simulink model "TrajectoryTracking_2015b_00"  (R2017a)
settings: Solver=ode45  StartTime=0.0  StopTime=125  RelTol=1e-3
values from neighbouring files (symbols this model uses):
  B_input = B_T    [ErrorDynamicsControllerDesign.m]
  tau_d_1 = C_RB1+C_A1+D1+G1    [DesiredInputOptimalConfiguration.m]
  tau_d_2 = C_RB2+C_A2+D2+G2    [DesiredInputOptimalConfiguration.m]
undefined symbols (not defined in the file or in its folder): angular_velocity_pitch_1, angular_velocity_pitch_2, angular_velocity_roll_1, angular_velocity_roll_2, angular_velocity_yaw_1, angular_velocity_yaw_2, K1, K2, linear_velocity_x_1, linear_velocity_x_2, linear_velocity_y_1, linear_velocity_y_2, linear_velocity_z_1, linear_velocity_z_2, pitch_angle_1, pitch_angle_2, roll_angle_1, roll_angle_2, t_1_last, t_e_1, t_e_2, tau_d_3, tau_d_4, tau_d_5, tau_d_6, tau_d_7, u_d_1, u_d_2, u_d_optimized, veh, x1, x2, y1, y2, yaw_angle_1, yaw_angle_2, z1, z2
undefined symbols (not defined in the file): b_T1_optimized, b_T2_optimized, b_T3_optimized, b_T4_optimized, b_T5_optimized, b_T6_optimized, d_T1_optimized, d_T2_optimized, d_T3_optimized, d_T4_optimized, d_T5_optimized, d_T6_optimized, r_T1_optimized, r_T2_optimized, r_T3_optimized, r_T4_optimized, r_T5_optimized, r_T6_optimized
libraries: sharedtransform x1, shared6dofsys x1
(part 2 of 2)

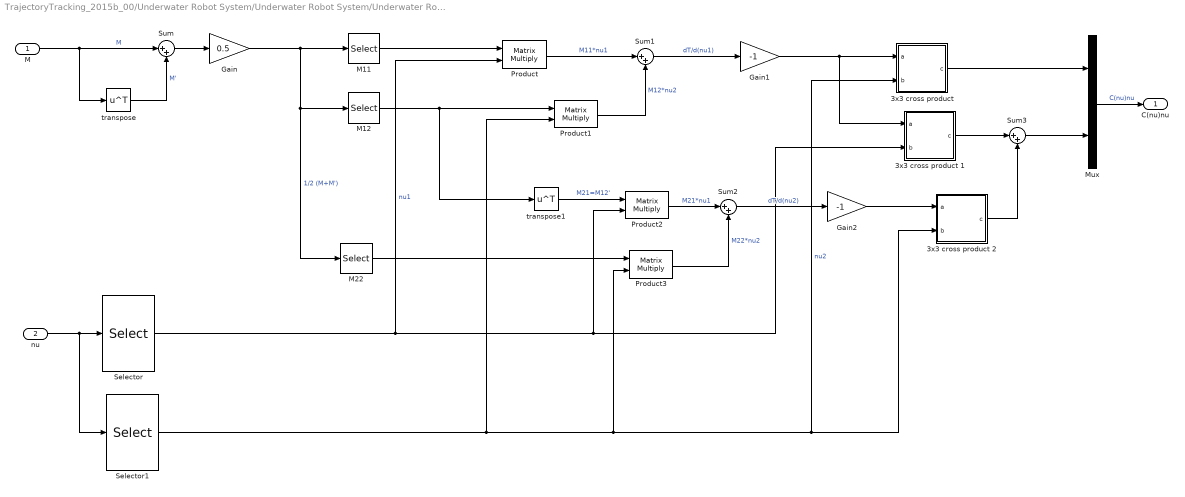
== system TrajectoryTracking_2015b_00/Underwater Robot System/Underwater Robot System/Underwater Robot Dynamics /6DOF Coriolis forces ==
  M : Inport
  nu : Inport  Port=2
  3x3 cross product : Subsystem
  3x3 cross product 1 : Subsystem
  3x3 cross product 2 : Subsystem
  Gain : Gain  Gain=0.5  SaturateOnIntegerOverflow=on  OutDataTypeStr=Inherit: Same as input  ParamDataTypeStr=Inherit: Same as input
  Gain1 : Gain  Gain=-1  SaturateOnIntegerOverflow=on  OutDataTypeStr=Inherit: Same as input  ParamDataTypeStr=Inherit: Same as input
  Gain2 : Gain  Gain=-1  SaturateOnIntegerOverflow=on  OutDataTypeStr=Inherit: Same as input  ParamDataTypeStr=Inherit: Same as input
  M11 : Selector  NumberOfDimensions=2  InputPortWidth=3  IndexOptions=Index vector (dialog),Index vector (dialog)  Indices=[1 2 3],[1 2 3]  OutputSizes=1
  M12 : Selector  NumberOfDimensions=2  InputPortWidth=3  IndexOptions=Index vector (dialog),Index vector (dialog)  Indices=[1 2 3],[4 5 6]  OutputSizes=1
  M22 : Selector  NumberOfDimensions=2  InputPortWidth=3  IndexOptions=Index vector (dialog),Index vector (dialog)  Indices=[4 5 6],[4 5 6]  OutputSizes=1
  Mux : Mux  Inputs=2
  Product{,1..3} (4 alike) : Product  Multiplication=Matrix(*)  SaturateOnIntegerOverflow=on  OutDataTypeStr=Inherit: Same as first input
  Selector : Selector  InputPortWidth=6  IndexOptions=Index vector (dialog)  Indices=[1 2 3]  OutputSizes=1
  Selector1 : Selector  InputPortWidth=6  IndexOptions=Index vector (dialog)  Indices=[4 5 6]  OutputSizes=1
  Sum{,1..3} (4 alike) : Sum  Inputs=|++  SaturateOnIntegerOverflow=on
  transpose : Math  Operator=transpose  SaturateOnIntegerOverflow=on
  transpose1 : Math  Operator=transpose  SaturateOnIntegerOverflow=on
  C(nu)nu : Outport
  wires:
  transpose/1 -> Sum/2  "M'"
  Sum/1 -> Gain/1
  Gain/1 -> M22/1, M12/1, M11/1  "1/2 (M+M')"
  Selector/1 -> Product2/2, 3x3 cross product 1/2(b), Product/2  "nu1"
  Selector1/1 -> 3x3 cross product/2(b), 3x3 cross product 2/2(b), Product3/2, Product1/2  "nu2"
  M11/1 -> Product/1
  Product/1 -> Sum1/1  "M11*nu1"
  M12/1 -> transpose1/1, Product1/1
  Product1/1 -> Sum1/2  "M12*nu2"
  Sum1/1 -> Gain1/1  "dT/d(nu1)"
  transpose1/1 -> Product2/1  "M21=M12'"
  Product2/1 -> Sum2/1  "M21*nu1"
  M22/1 -> Product3/1
  Product3/1 -> Sum2/2  "M22*nu2"
  Sum2/1 -> Gain2/1  "dT/d(nu2)"
  Gain1/1 -> 3x3 cross product/1(a), 3x3 cross product 1/1(a)
  3x3 cross product/1(c) -> Mux/1
  Gain2/1 -> 3x3 cross product 2/1(a)
  3x3 cross product 1/1(c) -> Sum3/1
  3x3 cross product 2/1(c) -> Sum3/2
  Sum3/1 -> Mux/2
  Mux/1 -> C(nu)nu/1  "C(nu)nu"
  nu/1 -> Selector/1, Selector1/1
  M/1 -> transpose/1, Sum/1  "M"

== system TrajectoryTracking_2015b_00/Nonlinear Transformation/Position Error /Nonlinear Orientation Transformation/pitch_error/theta_d ==
  SwitchSchedule : Inport
  1-D Lookup Table1 : Lookup_n-D  NumberOfTableDimensions=1  BreakpointsForDimension1=t_e_2  Table=pitch_angle_2  InternalRulePriority=Speed  RndMeth=Simplest  InputSameDT=on
  1-D Lookup Table3 : Lookup_n-D  NumberOfTableDimensions=1  BreakpointsForDimension1=t_e_1  Table=pitch_angle_1  InternalRulePriority=Speed  RndMeth=Simplest  InputSameDT=on
  Add : Sum  Inputs=+-
  Clock : Clock
  Constant : Constant  Value=t_1_last
  Multiport Switch1 : MultiPortSwitch  Inputs=2
  Transfer Fcn : TransferFcn  Denominator=[1.5 1]
  theta_d : Outport
  wires:
  SwitchSchedule/1 -> Multiport Switch1/1
  1-D Lookup Table1/1 -> Multiport Switch1/3
  1-D Lookup Table3/1 -> Multiport Switch1/2
  Constant/1 -> Add/2
  Multiport Switch1/1 -> Transfer Fcn/1
  Clock/1 -> Add/1, 1-D Lookup Table3/1
  Add/1 -> 1-D Lookup Table1/1
  Transfer Fcn/1 -> theta_d/1

== system TrajectoryTracking_2015b_00/Nonlinear Transformation/Position Error /Nonlinear Orientation Transformation/roll_error/phi_d ==
  SwitchSchedule : Inport
  1-D Lookup Table1 : Lookup_n-D  NumberOfTableDimensions=1  BreakpointsForDimension1=t_e_2  Table=roll_angle_2  InternalRulePriority=Speed  RndMeth=Simplest  InputSameDT=on
  1-D Lookup Table3 : Lookup_n-D  NumberOfTableDimensions=1  BreakpointsForDimension1=t_e_1  Table=roll_angle_1  InternalRulePriority=Speed  RndMeth=Simplest  InputSameDT=on
  Add : Sum  Inputs=+-
  Clock : Clock
  Constant : Constant  Value=t_1_last
  Multiport Switch : MultiPortSwitch  Inputs=2
  Transfer Fcn : TransferFcn  Denominator=[1 1]
  phi_d : Outport
  wires:
  1-D Lookup Table1/1 -> Multiport Switch/3
  1-D Lookup Table3/1 -> Multiport Switch/2
  Constant/1 -> Add/2
  Multiport Switch/1 -> Transfer Fcn/1
  Clock/1 -> Add/1, 1-D Lookup Table3/1
  Add/1 -> 1-D Lookup Table1/1
  SwitchSchedule/1 -> Multiport Switch/1
  Transfer Fcn/1 -> phi_d/1

== system TrajectoryTracking_2015b_00/Nonlinear Transformation/Position Error /Nonlinear Orientation Transformation/yaw_error/theta_d ==
  SwitchSchedule : Inport
  1-D Lookup Table1 : Lookup_n-D  NumberOfTableDimensions=1  BreakpointsForDimension1=t_e_2  Table=yaw_angle_2  InternalRulePriority=Speed  RndMeth=Simplest  InputSameDT=on
  1-D Lookup Table3 : Lookup_n-D  NumberOfTableDimensions=1  BreakpointsForDimension1=t_e_1  Table=yaw_angle_1  InternalRulePriority=Speed  RndMeth=Simplest  InputSameDT=on
  Add : Sum  Inputs=+-
  Clock : Clock
  Constant : Constant  Value=t_1_last
  Multiport Switch1 : MultiPortSwitch  Inputs=2
  Transfer Fcn : TransferFcn  Denominator=[1 1]
  yaw_d : Outport
  wires:
  SwitchSchedule/1 -> Multiport Switch1/1
  1-D Lookup Table1/1 -> Multiport Switch1/3
  1-D Lookup Table3/1 -> Multiport Switch1/2
  Constant/1 -> Add/2
  Multiport Switch1/1 -> Transfer Fcn/1
  Clock/1 -> Add/1, 1-D Lookup Table3/1
  Add/1 -> 1-D Lookup Table1/1
  Transfer Fcn/1 -> yaw_d/1

== system TrajectoryTracking_2015b_00/Nonlinear Transformation/Position Error /Nonlinear Position Transformation/x_error/x_d ==
  SwitchSchedule : Inport
  1-D Lookup Table7 : Lookup_n-D  NumberOfTableDimensions=1  BreakpointsForDimension1=t_e_2  Table=x2  InternalRulePriority=Speed  RndMeth=Simplest  InputSameDT=on
  1-D Lookup Table9 : Lookup_n-D  NumberOfTableDimensions=1  BreakpointsForDimension1=t_e_1  Table=x1  InternalRulePriority=Speed  RndMeth=Simplest  InputSameDT=on
  Add : Sum  Inputs=+-
  Clock : Clock
  Constant : Constant  Value=t_1_last
  Multiport Switch1 : MultiPortSwitch  Inputs=2
  Transfer Fcn1 : TransferFcn  Denominator=[1 1]
  x_d : Outport
  wires:
  1-D Lookup Table7/1 -> Multiport Switch1/3
  1-D Lookup Table9/1 -> Multiport Switch1/2
  Constant/1 -> Add/2
  Multiport Switch1/1 -> Transfer Fcn1/1
  SwitchSchedule/1 -> Multiport Switch1/1
  Add/1 -> 1-D Lookup Table7/1
  Transfer Fcn1/1 -> x_d/1
  Clock/1 -> Add/1, 1-D Lookup Table9/1

== system TrajectoryTracking_2015b_00/Nonlinear Transformation/Position Error /Nonlinear Position Transformation/y_error/y_d ==
  SwitchSchedule : Inport
  1-D Lookup Table10 : Lookup_n-D  NumberOfTableDimensions=1  BreakpointsForDimension1=t_e_1  Table=y1  InternalRulePriority=Speed  RndMeth=Simplest  InputSameDT=on
  1-D Lookup Table8 : Lookup_n-D  NumberOfTableDimensions=1  BreakpointsForDimension1=t_e_2  Table=y2  InternalRulePriority=Speed  RndMeth=Simplest  InputSameDT=on
  Add : Sum  Inputs=+-
  Clock : Clock
  Constant : Constant  Value=t_1_last
  Multiport Switch : MultiPortSwitch  Inputs=2
  Transfer Fcn : TransferFcn  Denominator=[1 1]
  y_d : Outport
  wires:
  1-D Lookup Table8/1 -> Multiport Switch/3
  1-D Lookup Table10/1 -> Multiport Switch/2
  Constant/1 -> Add/2
  Multiport Switch/1 -> Transfer Fcn/1
  Add/1 -> 1-D Lookup Table8/1
  SwitchSchedule/1 -> Multiport Switch/1
  Clock/1 -> Add/1, 1-D Lookup Table10/1
  Transfer Fcn/1 -> y_d/1

== system TrajectoryTracking_2015b_00/Nonlinear Transformation/Position Error /Nonlinear Position Transformation/z_error/z_d ==
  SwitchSchedule : Inport
  1-D Lookup Table1 : Lookup_n-D  NumberOfTableDimensions=1  BreakpointsForDimension1=t_e_2  Table=z2  InternalRulePriority=Speed  RndMeth=Simplest  InputSameDT=on
  1-D Lookup Table3 : Lookup_n-D  NumberOfTableDimensions=1  BreakpointsForDimension1=t_e_1  Table=z1  InternalRulePriority=Speed  RndMeth=Simplest  InputSameDT=on
  Add : Sum  Inputs=+-
  Clock : Clock
  Constant2 : Constant  Value=t_1_last
  Multiport Switch : MultiPortSwitch  Inputs=2
  Transfer Fcn : TransferFcn  Denominator=[1 1]
  z_d : Outport
  wires:
  1-D Lookup Table1/1 -> Multiport Switch/3
  1-D Lookup Table3/1 -> Multiport Switch/2
  Constant2/1 -> Add/2
  Multiport Switch/1 -> Transfer Fcn/1
  Add/1 -> 1-D Lookup Table1/1
  SwitchSchedule/1 -> Multiport Switch/1
  Clock/1 -> Add/1, 1-D Lookup Table3/1
  Transfer Fcn/1 -> z_d/1

== system TrajectoryTracking_2015b_00/Underwater Robot System/Underwater Robot System/Underwater Robot Dynamics /6DOF Coriolis forces/3x3 cross product ==
  a : Inport
  b : Inport  Port=2
  Product : Product  SaturateOnIntegerOverflow=on  InputSameDT=on  OutDataTypeStr=Inherit: Same as first input
  Product1 : Product  SaturateOnIntegerOverflow=on  InputSameDT=on  OutDataTypeStr=Inherit: Same as first input
  Selector : Selector  InputPortWidth=3  IndexOptions=Index vector (dialog)  Indices=[2 3 1]  OutputSizes=1
  Selector1 : Selector  InputPortWidth=3  IndexOptions=Index vector (dialog)  Indices=[3 1 2]  OutputSizes=1
  Selector2 : Selector  InputPortWidth=3  IndexOptions=Index vector (dialog)  Indices=[2 3 1]  OutputSizes=1
  Selector3 : Selector  InputPortWidth=3  IndexOptions=Index vector (dialog)  Indices=[3 1 2]  OutputSizes=1
  Sum : Sum  Inputs=+|-  SaturateOnIntegerOverflow=on  InputSameDT=on  OutDataTypeStr=Inherit: Same as first input
  c : Outport  InitialOutput=0
  wires:
  Selector3/1 -> Product1/1
  Selector2/1 -> Product1/2
  Product1/1 -> Sum/2
  Selector1/1 -> Product/2
  Product/1 -> Sum/1
  a/1 -> Selector3/1, Selector/1
  Selector/1 -> Product/1
  b/1 -> Selector2/1, Selector1/1
  Sum/1 -> c/1

== system TrajectoryTracking_2015b_00/Underwater Robot System/Underwater Robot System/Underwater Robot Dynamics /6DOF Coriolis forces/3x3 cross product 1 ==
  a : Inport
  b : Inport  Port=2
  Product : Product  SaturateOnIntegerOverflow=on  InputSameDT=on  OutDataTypeStr=Inherit: Same as first input
  Product1 : Product  SaturateOnIntegerOverflow=on  InputSameDT=on  OutDataTypeStr=Inherit: Same as first input
  Selector : Selector  InputPortWidth=3  IndexOptions=Index vector (dialog)  Indices=[2 3 1]  OutputSizes=1
  Selector1 : Selector  InputPortWidth=3  IndexOptions=Index vector (dialog)  Indices=[3 1 2]  OutputSizes=1
  Selector2 : Selector  InputPortWidth=3  IndexOptions=Index vector (dialog)  Indices=[2 3 1]  OutputSizes=1
  Selector3 : Selector  InputPortWidth=3  IndexOptions=Index vector (dialog)  Indices=[3 1 2]  OutputSizes=1
  Sum : Sum  Inputs=+|-  SaturateOnIntegerOverflow=on  InputSameDT=on  OutDataTypeStr=Inherit: Same as first input
  c : Outport  InitialOutput=0
  wires:
  Selector3/1 -> Product1/1
  Selector2/1 -> Product1/2
  Product1/1 -> Sum/2
  Selector1/1 -> Product/2
  Product/1 -> Sum/1
  a/1 -> Selector3/1, Selector/1
  Selector/1 -> Product/1
  b/1 -> Selector2/1, Selector1/1
  Sum/1 -> c/1

== system TrajectoryTracking_2015b_00/Underwater Robot System/Underwater Robot System/Underwater Robot Dynamics /6DOF Coriolis forces/3x3 cross product 2 ==
  a : Inport
  b : Inport  Port=2
  Product : Product  SaturateOnIntegerOverflow=on  InputSameDT=on  OutDataTypeStr=Inherit: Same as first input
  Product1 : Product  SaturateOnIntegerOverflow=on  InputSameDT=on  OutDataTypeStr=Inherit: Same as first input
  Selector : Selector  InputPortWidth=3  IndexOptions=Index vector (dialog)  Indices=[2 3 1]  OutputSizes=1
  Selector1 : Selector  InputPortWidth=3  IndexOptions=Index vector (dialog)  Indices=[3 1 2]  OutputSizes=1
  Selector2 : Selector  InputPortWidth=3  IndexOptions=Index vector (dialog)  Indices=[2 3 1]  OutputSizes=1
  Selector3 : Selector  InputPortWidth=3  IndexOptions=Index vector (dialog)  Indices=[3 1 2]  OutputSizes=1
  Sum : Sum  Inputs=+|-  SaturateOnIntegerOverflow=on  InputSameDT=on  OutDataTypeStr=Inherit: Same as first input
  c : Outport  InitialOutput=0
  wires:
  Selector3/1 -> Product1/1
  Selector2/1 -> Product1/2
  Product1/1 -> Sum/2
  Selector1/1 -> Product/2
  Product/1 -> Sum/1
  a/1 -> Selector3/1, Selector/1
  Selector/1 -> Product/1
  b/1 -> Selector2/1, Selector1/1
  Sum/1 -> c/1

== matlab function TrajectoryTracking_2015b_00/Switch Control ==
  data: u input; y output
function y = SwitchSchedule(u)
%% in this function 
if(u>=100 && u<=125)
    y=2;
else
    y=1;
end
